simulink model "MODELL_aktiver_Stabi"  (R2016a)
settings: Solver=ode4  StartTime=0.0  StopTime=10  FixedStep=0.001  RelTol=1e-3
undefined symbols (not defined in the file): A_Kolben, b_d, b_f, b_r, b_s, c, c_R, d, d_R, G, g, h_Aktor, h_S_DZ, h_Stabi, I_p_Stabi, J_x_A, J_x_F, m_A, m_F, m_R, sigbuilder_block
settings Model: Creator=Michaél  LastModifiedBy=Michaél

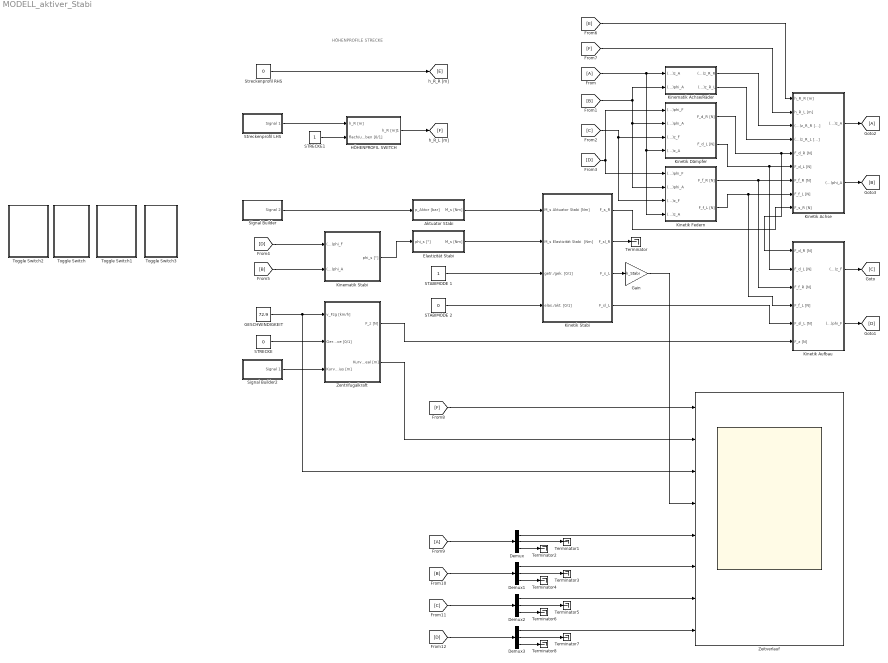
== system MODELL_aktiver_Stabi ==
  note: HÖHENPROFILE
      | STRECKE
  Aktuator Stabi : Subsystem
  Demux{,1..3} (4 alike) : Demux  Outputs=3
  Elastizität Stabi : Subsystem
  GESCHWINDIGKEIT : Constant  Value=72.9
  Gain : Gain  Gain=h_Stabi
  HÖHENPROFIL SWITCH : Subsystem
  Kinematik Achse/Räder : Subsystem
  Kinematik Stabi : Subsystem
  Kinetik Achse : Subsystem
  Kinetik Aufbau : Subsystem
  Kinetik Dämpfer : Subsystem
  Kinetik Federn : Subsystem
  Kinetik Stabi : Subsystem
  STABIMODE 1 : Constant
  STABIMODE 2 : Constant  Value=0
  STRECKE : Constant  Value=0
  STRECKE1 : Constant
  Signal Builder : Subsystem  Tag=STV Subsys  LoadFcn=sigbuilder_block('load');  StartFcn=sigbuilder_block('start');  StopFcn=sigbuilder_block('stop');  ClipboardFcn=sigbuilder_block('clipboard');  mask(Sigbuilder block){}
      mask help: Simulink:masks:SigbuilderBlock_MD
      mask init:
      | if ~strcmp(get_param(bdroot(gcbh),'SimulationStatus'),'stopped') tuvar = sigbuilder_block('maskInit'); end
      settings: CopyFcn=sigbuilder_block('copy');  DeleteFcn=sigbuilder_block('delete');  ModelCloseFcn=sigbuilder_block('modelClose');  PreSaveFcn=sigbuilder_block('preSave');  PauseFcn=sigbuilder_block('pause');  ContinueFcn=sigbuilder_block('continue');  NameChangeFcn=sigbuilder_block('namechange');  OpenFcn=sigbuilder_block('open',[437.25 153 550.5 359.25 ]);  CloseFcn=sigbuilder_block('close');
      mask Display: plot(0, 0, 100, 100,[2, 2, 32, 32, 2], [68, 8, 8, 68, 68],[32, 2], [38, 38], [32, 19, 2],[53, 60, 44], [32, 17, 17, 2],[16, 16, 31, 31]);txt = getActiveGroup(gcbh);text(2, 100, txt,'verticalAlignment', 'top');
  Signal Builder2 : Subsystem  Tag=STV Subsys  LoadFcn=sigbuilder_block('load');  StartFcn=sigbuilder_block('start');  StopFcn=sigbuilder_block('stop');  ClipboardFcn=sigbuilder_block('clipboard');  mask(Sigbuilder block){}
      mask help: Simulink:masks:SigbuilderBlock_MD
      mask init:
      | if ~strcmp(get_param(bdroot(gcbh),'SimulationStatus'),'stopped') tuvar = sigbuilder_block('maskInit'); end
      settings: CopyFcn=sigbuilder_block('copy');  DeleteFcn=sigbuilder_block('delete');  ModelCloseFcn=sigbuilder_block('modelClose');  PreSaveFcn=sigbuilder_block('preSave');  PauseFcn=sigbuilder_block('pause');  ContinueFcn=sigbuilder_block('continue');  NameChangeFcn=sigbuilder_block('namechange');  OpenFcn=sigbuilder_block('open',[437.25 153 550.5 359.25 ]);  CloseFcn=sigbuilder_block('close');
      mask Display: plot(0, 0, 100, 100,[2, 2, 32, 32, 2], [68, 8, 8, 68, 68],[32, 2], [38, 38], [32, 19, 2],[53, 60, 44], [32, 17, 17, 2],[16, 16, 31, 31]);txt = getActiveGroup(gcbh);text(2, 100, txt,'verticalAlignment', 'top');
  Streckenprofil LHS : Subsystem  Tag=STV Subsys  LoadFcn=sigbuilder_block('load');  StartFcn=sigbuilder_block('start');  StopFcn=sigbuilder_block('stop');  ClipboardFcn=sigbuilder_block('clipboard');  mask(Sigbuilder block){}
      mask help: Simulink:masks:SigbuilderBlock_MD
      mask init:
      | if ~strcmp(get_param(bdroot(gcbh),'SimulationStatus'),'stopped') tuvar = sigbuilder_block('maskInit'); end
      settings: CopyFcn=sigbuilder_block('copy');  DeleteFcn=sigbuilder_block('delete');  ModelCloseFcn=sigbuilder_block('modelClose');  PreSaveFcn=sigbuilder_block('preSave');  PauseFcn=sigbuilder_block('pause');  ContinueFcn=sigbuilder_block('continue');  NameChangeFcn=sigbuilder_block('namechange');  OpenFcn=sigbuilder_block('open',[437.25 153 550.5 359.25 ]);  CloseFcn=sigbuilder_block('close');
      mask Display: plot(0, 0, 100, 100,[2, 2, 32, 32, 2], [68, 8, 8, 68, 68],[32, 2], [38, 38], [32, 19, 2],[53, 60, 44], [32, 17, 17, 2],[16, 16, 31, 31]);txt = getActiveGroup(gcbh);text(2, 100, txt,'verticalAlignment', 'top');
  Streckenprofil RHS : Constant  Value=0
  Terminator{,1..8} (9 alike) : Terminator
  Toggle Switch : Subsystem  DialogController=hmiCreateDDGDialog  IsWebBlock=on  mask(MWDashboardBlock){webBlockId=3030378f-6338-4f5a-b9a6-65f9c6752063, webBlockType=toggleswitch, ShowInLibBrowser=on, ShowInitialText=on, HMISrcModelName=MODELL_aktiver_Stabi_OPENME}
      mask prompts: webBlockId "WebBlock Id"; webBlockType "WebBlock Type"; HMISrcModelName "Source Model"
      mask help: Set on/off value to tune parameters or variables.
      mask Help: helpview([docroot '/mapfiles/simulink.map'], 'hmi_switch')
      mask Display:
      | if strcmp(get_param(bdroot(gcb),'BlockDiagramType'),'library')
      |  image([(matlabroot) '/toolbox/simulink/hmi/icons/ToggleSwitch.png'])
      | end
  Toggle Switch1 : Subsystem  DialogController=hmiCreateDDGDialog  IsWebBlock=on  mask(MWDashboardBlock){webBlockId=66d0c5f1-b412-4773-8f90-b24a010b2d54, webBlockType=toggleswitch, ShowInLibBrowser=on, ShowInitialText=on, HMISrcModelName=MODELL_aktiver_Stabi_OPENME}
      mask prompts: webBlockId "WebBlock Id"; webBlockType "WebBlock Type"; HMISrcModelName "Source Model"
      mask help: Set on/off value to tune parameters or variables.
      mask Help: helpview([docroot '/mapfiles/simulink.map'], 'hmi_switch')
      mask Display:
      | if strcmp(get_param(bdroot(gcb),'BlockDiagramType'),'library')
      |  image([(matlabroot) '/toolbox/simulink/hmi/icons/ToggleSwitch.png'])
      | end
  Toggle Switch2 : Subsystem  DialogController=hmiCreateDDGDialog  IsWebBlock=on  mask(MWDashboardBlock){webBlockId=f8bafa90-b455-434b-b4c4-d0f007b97158, webBlockType=toggleswitch, ShowInLibBrowser=on, ShowInitialText=on, HMISrcModelName=MODELL_aktiver_Stabi_OPENME}
      mask prompts: webBlockId "WebBlock Id"; webBlockType "WebBlock Type"; HMISrcModelName "Source Model"
      mask help: Set on/off value to tune parameters or variables.
      mask Help: helpview([docroot '/mapfiles/simulink.map'], 'hmi_switch')
      mask Display:
      | if strcmp(get_param(bdroot(gcb),'BlockDiagramType'),'library')
      |  image([(matlabroot) '/toolbox/simulink/hmi/icons/ToggleSwitch.png'])
      | end
  Toggle Switch3 : Subsystem  DialogController=hmiCreateDDGDialog  IsWebBlock=on  mask(MWDashboardBlock){webBlockId=5b0afa38-ed08-4fc5-84e4-437145695883, webBlockType=toggleswitch, ShowInLibBrowser=on, ShowInitialText=on, HMISrcModelName=MODELL_aktiver_Stabi_OPENME}
      mask prompts: webBlockId "WebBlock Id"; webBlockType "WebBlock Type"; HMISrcModelName "Source Model"
      mask help: Set on/off value to tune parameters or variables.
      mask Help: helpview([docroot '/mapfiles/simulink.map'], 'hmi_switch')
      mask Display:
      | if strcmp(get_param(bdroot(gcb),'BlockDiagramType'),'library')
      |  image([(matlabroot) '/toolbox/simulink/hmi/icons/ToggleSwitch.png'])
      | end
  Zeitverlauf : Scope  NumInputPorts=8
  Zentrifugalkraft : Subsystem
  wires:
  Aktuator Stabi/1(M_s [Nm]) -> Kinetik Stabi/1(M_s Aktuator Stabi [Nm])
  Kinetik Stabi/2(F_sl_R) -> Terminator/1
  Kinetik Federn/1(F_f_R [N]) -> Kinetik Aufbau/3(F_f_R [N]), Kinetik Achse/7(F_f_R [N])
  Kinetik Federn/2(F_f_L [N]) -> Kinetik Aufbau/4(F_f_L [N]), Kinetik Achse/8(F_f_L [N])
  Kinetik Dämpfer/1(F_d_R [N]) -> Kinetik Aufbau/1(F_d_R [N]), Kinetik Achse/5(F_d_R [N])
  Kinetik Dämpfer/2(F_d_L [N]) -> Kinetik Aufbau/2(F_d_L [N]), Kinetik Achse/6(F_d_L [N])
  Kinetik Stabi/3(F_s_L) -> Gain/1
  Zentrifugalkraft/1(F_z [N]) -> Kinetik Aufbau/6("F_z [N] ")
  Kinematik Stabi/1(phi_s [°]) -> Elastizität Stabi/1(phi_s [°])
  Kinematik Achse/Räder/1((...)z_R_R) -> Kinetik Achse/3((...)z_R_R [...])
  Kinematik Achse/Räder/2((...)z_R_L) -> Kinetik Achse/4((...)z_R_L [...])
  Kinetik Aufbau/1((...)z_F) -> [C]
  Kinetik Aufbau/2((...)phi_F) -> [D]
  Kinetik Achse/1((...)z_A) -> [A]
  Kinetik Achse/2((...)phi_A) -> [B]
  [A] -> Kinetik Federn/4((...)z_A), Kinetik Dämpfer/4((...)z_A), Kinematik Achse/Räder/1((...)z_A)
  [B] -> Kinetik Federn/2((...)phi_A), Kinetik Dämpfer/2((...)phi_A), Kinematik Achse/Räder/2((...)phi_A)
  [C] -> Kinetik Dämpfer/3((...)z_F), Kinetik Federn/3((...)z_F)
  [D] -> Kinetik Federn/1((...)phi_F), Kinetik Dämpfer/1((...)phi_F)
  [D] -> Kinematik Stabi/1((...)phi_F)
  [B] -> Kinematik Stabi/2((...)phi_A)
  STABIMODE 1/1 -> Kinetik Stabi/3("getr./gek. [0/1] ")
  STRECKE/1 -> Zentrifugalkraft/2(Gerade/Kurve [0/1])
  STABIMODE 2/1 -> Kinetik Stabi/4("elas./akt. [0/1] ")
  [E] -> Kinetik Achse/1(h_R_R [m])
  [F] -> Kinetik Achse/2(h_R_L [m])
  Signal Builder/1(Signal 2) -> Aktuator Stabi/1(p_Aktor [bar])
  Signal Builder2/1(Signal 1) -> Zentrifugalkraft/3(Kurvenradius [m])
  [F] -> Zeitverlauf/1
  GESCHWINDIGKEIT/1 -> Zeitverlauf/3, Zentrifugalkraft/1(v_Fzg [km/h])
  [A] -> Demux/1
  Demux/1 -> Zeitverlauf/5
  [B] -> Demux1/1
  Demux1/1 -> Zeitverlauf/6
  [C] -> Demux2/1
  Demux2/1 -> Zeitverlauf/7
  [D] -> Demux3/1
  Elastizität Stabi/1(M_s [Nm]) -> Kinetik Stabi/2(M_s Elastizität Stabi  [Nm])
  Gain/1 -> Zeitverlauf/4
  Kinetik Stabi/1(F_s_R) -> Kinetik Achse/9(F_s_R [N])
  Kinetik Stabi/4(F_sl_L) -> Kinetik Aufbau/5("F_sl_L [N] ")
  Streckenprofil RHS/1 -> [E]
  Streckenprofil LHS/1(Signal 1) -> HÖHENPROFIL SWITCH/1(h_R [m])
  HÖHENPROFIL SWITCH/1(h_R [m]1) -> [F]
  STRECKE1/1 -> HÖHENPROFIL SWITCH/2(flach/uneben [0/1])
  Demux3/1 -> Zeitverlauf/8
  Demux/2 -> Terminator1/1
  Demux/3 -> Terminator2/1
  Demux1/2 -> Terminator3/1
  Demux1/3 -> Terminator4/1
  Demux2/2 -> Terminator5/1
  Demux2/3 -> Terminator6/1
  Demux3/2 -> Terminator7/1
  Demux3/3 -> Terminator8/1
  Zentrifugalkraft/2(Kurvenradius real [m]) -> Zeitverlauf/2

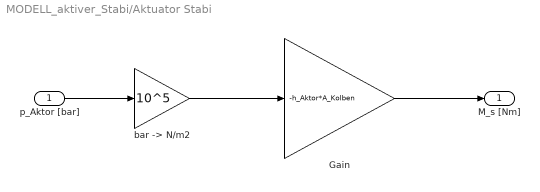
== system MODELL_aktiver_Stabi/Aktuator Stabi ==
  p_Aktor [bar] : Inport
  Gain : Gain  Gain=-h_Aktor*A_Kolben
  "bar -> N/m2" : Gain  Gain=10^5
  M_s [Nm] : Outport
  wires:
  Gain/1 -> M_s [Nm]/1
  p_Aktor [bar]/1 -> "bar -> N/m2"/1
  "bar -> N/m2"/1 -> Gain/1

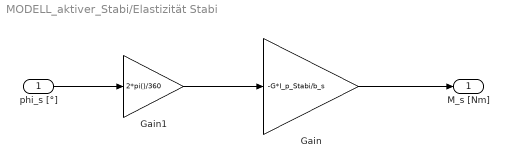
== system MODELL_aktiver_Stabi/Elastizität Stabi ==
  phi_s [°] : Inport
  Gain : Gain  Gain=-G*I_p_Stabi/b_s
  Gain1 : Gain  Gain=2*pi()/360
  M_s [Nm] : Outport
  wires:
  phi_s [°]/1 -> Gain1/1
  Gain1/1 -> Gain/1
  Gain/1 -> M_s [Nm]/1

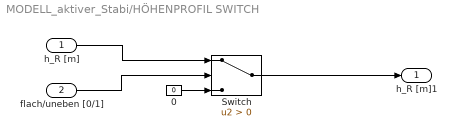
== system MODELL_aktiver_Stabi/HÖHENPROFIL SWITCH ==
  h_R [m] : Inport
  flach/uneben [0/1] : Inport  Port=2
  0 : Constant  Value=0
  Switch : Switch  Criteria=u2 > Threshold
  h_R [m]1 : Outport
  wires:
  h_R [m]/1 -> Switch/1
  Switch/1 -> h_R [m]1/1
  flach/uneben [0/1]/1 -> Switch/2
  0/1 -> Switch/3

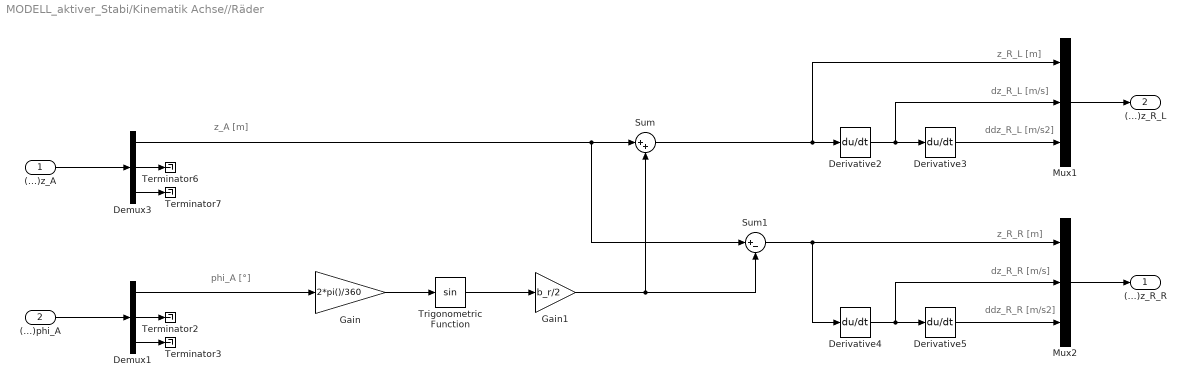
== system MODELL_aktiver_Stabi/Kinematik Achse//Räder ==
  note: z_R_L [m]
  note: dz_R_L [m/s]
  note: ddz_R_L [m/s2]
  note: z_R_R [m]
  note: dz_R_R [m/s]
  note: ddz_R_R [m/s2]
  note: z_A [m]
  note: phi_A [°]
  (...)z_A : Inport
  (...)phi_A : Inport  Port=2
  Demux1 : Demux  Outputs=3
  Demux3 : Demux  Outputs=3
  Derivative{2..5} (4 alike) : Derivative
  Gain : Gain  Gain=2*pi()/360
  Gain1 : Gain  Gain=b_r/2
  Mux1 : Mux  Inputs=3
  Mux2 : Mux  Inputs=3
  Sum : Sum  Inputs=|++
  Sum1 : Sum  Inputs=|+-
  Terminator{2..3,6..7} (4 alike) : Terminator
  Trigonometric Function : Trigonometry
  (...)z_R_R : Outport
  (...)z_R_L : Outport  Port=2
  wires:
  Gain/1 -> Trigonometric Function/1
  Trigonometric Function/1 -> Gain1/1
  Demux1/1 -> Gain/1
  Demux3/1 -> Sum1/1, Sum/1
  Gain1/1 -> Sum1/2, Sum/2
  Derivative3/1 -> Mux1/3
  Derivative2/1 -> Mux1/2, Derivative3/1
  Sum/1 -> Mux1/1, Derivative2/1
  Mux1/1 -> (...)z_R_L/1
  Derivative5/1 -> Mux2/3
  Derivative4/1 -> Mux2/2, Derivative5/1
  Sum1/1 -> Derivative4/1, Mux2/1
  Mux2/1 -> (...)z_R_R/1
  (...)z_A/1 -> Demux3/1
  Demux3/3 -> Terminator7/1
  Demux3/2 -> Terminator6/1
  (...)phi_A/1 -> Demux1/1
  Demux1/3 -> Terminator3/1
  Demux1/2 -> Terminator2/1

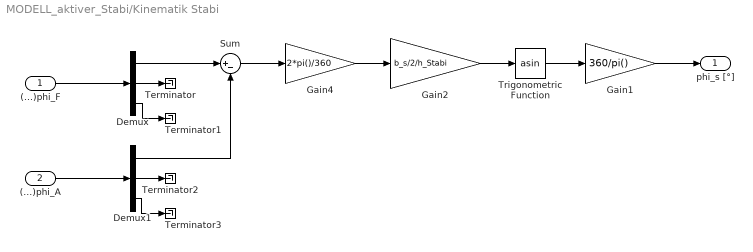
== system MODELL_aktiver_Stabi/Kinematik Stabi ==
  (...)phi_F : Inport
  (...)phi_A : Inport  Port=2
  Demux : Demux  Outputs=3
  Demux1 : Demux  Outputs=3
  Gain1 : Gain  Gain=360/pi()
  Gain2 : Gain  Gain=b_s/2/h_Stabi
  Gain4 : Gain  Gain=2*pi()/360
  Sum : Sum  Inputs=|+-
  Terminator{,1..3} (4 alike) : Terminator
  Trigonometric Function : Trigonometry  Operator=asin
  phi_s [°] : Outport
  wires:
  Sum/1 -> Gain4/1
  (...)phi_F/1 -> Demux/1
  (...)phi_A/1 -> Demux1/1
  Demux/1 -> Sum/1
  Demux1/1 -> Sum/2
  Demux/2 -> Terminator/1
  Demux/3 -> Terminator1/1
  Demux1/3 -> Terminator3/1
  Demux1/2 -> Terminator2/1
  Gain2/1 -> Trigonometric Function/1
  Gain1/1 -> phi_s [°]/1
  Gain4/1 -> Gain2/1
  Trigonometric Function/1 -> Gain1/1

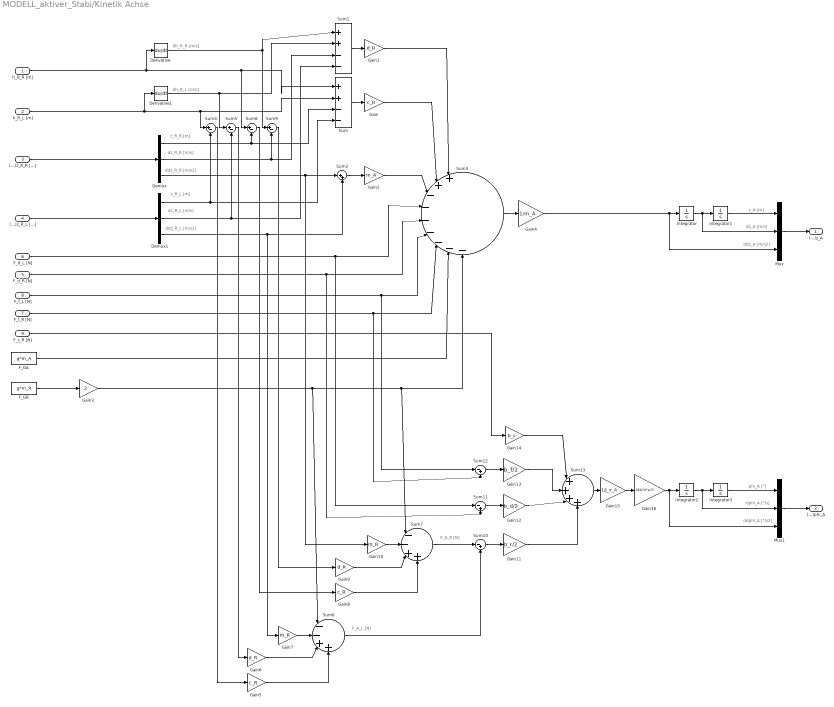
== system MODELL_aktiver_Stabi/Kinetik Achse ==
  note: F_A_L [N]
  note: dh_R_L [m/s]
  note: dh_R_R [m/s]
  note: z_R_L [m]
  note: dz_R_L [m/s]
  note: ddz_R_L [m/s2]
  note: z_R_R [m]
  note: dz_R_R [m/s]
  note: ddz_R_R [m/s2]
  note: z_A [m]
  note: dz_A [m/s]
  note: ddz_A [m/s2]
  note: F_A_R [N]
  note: phi_A [°]
  note: dphi_A [°/s]
  note: ddphi_A [°/s2]
  h_R_R [m] : Inport
  h_R_L [m] : Inport  Port=2
  (...)z_R_R [...] : Inport  Port=3
  (...)z_R_L [...] : Inport  Port=4
  F_d_R [N] : Inport  Port=5
  F_d_L [N] : Inport  Port=6
  F_f_R [N] : Inport  Port=7
  F_f_L [N] : Inport  Port=8
  F_s_R [N] : Inport  Port=9
  Demux : Demux  Outputs=3
  Demux1 : Demux  Outputs=3
  Derivative : Derivative
  Derivative1 : Derivative
  F_GA : Constant  Value=g*m_A
  F_GR : Constant  Value=g*m_R
  Gain : Gain  Gain=c_R
  Gain1 : Gain  Gain=d_R
  Gain10 : Gain  Gain=m_R
  Gain11 : Gain  Gain=b_r/2
  Gain12 : Gain  Gain=b_d/2
  Gain13 : Gain  Gain=b_f/2
  Gain14 : Gain  Gain=b_s
  Gain15 : Gain  Gain=1/J_x_A
  Gain16 : Gain  Gain=360/(2*pi())
  Gain2 : Gain  Gain=m_A
  Gain3 : Gain  Gain=2
  Gain4 : Gain  Gain=1/m_A
  Gain5 : Gain  Gain=c_R
  Gain6 : Gain  Gain=d_R
  Gain7 : Gain  Gain=m_R
  Gain8 : Gain  Gain=c_R
  Gain9 : Gain  Gain=d_R
  Integrator : Integrator
  Integrator1 : Integrator  InitialCondition=-0.03
  Integrator2 : Integrator
  Integrator3 : Integrator
  Mux : Mux  Inputs=3
  Mux1 : Mux  Inputs=3
  Sum : Sum  Inputs=|++--
  Sum1 : Sum  Inputs=|++--
  Sum10 : Sum  Inputs=|-+
  Sum11 : Sum  Inputs=|-+
  Sum12 : Sum  Inputs=|-+
  Sum13 : Sum  Inputs=|++++
  Sum2 : Sum  Inputs=|++
  Sum3 : Sum  Inputs=|++-------
  Sum{4..5,8..9} (4 alike) : Sum  Inputs=|+-
  Sum6 : Sum  Inputs=|--++
  Sum7 : Sum  Inputs=|--++
  (...)z_A : Outport
  (...)phi_A : Outport  Port=2
  wires:
  (...)z_R_R [...]/1 -> Demux/1
  (...)z_R_L [...]/1 -> Demux1/1
  h_R_R [m]/1 -> Sum8/1, Sum/1, Derivative/1
  h_R_L [m]/1 -> Sum4/1, Sum/2, Derivative1/1
  Demux/1 -> Sum8/2, Sum/3
  Demux1/1 -> Sum/4, Sum4/2
  Sum/1 -> Gain/1
  Derivative/1 -> Sum9/1, Sum1/1
  Derivative1/1 -> Sum1/2, Sum5/1
  Demux1/2 -> Sum1/4, Sum5/2
  Demux1/3 -> Sum2/2, Gain7/1
  Sum1/1 -> Gain1/1
  Sum2/1 -> Gain2/1
  F_GR/1 -> Gain3/1
  Gain1/1 -> Sum3/1
  Gain/1 -> Sum3/2
  Gain2/1 -> Sum3/3
  F_d_R [N]/1 -> Sum3/5, Sum11/2
  F_f_L [N]/1 -> Sum12/1, Sum3/6
  F_GA/1 -> Sum3/8
  Gain3/1 -> Sum3/9, Sum7/1, Sum6/1
  Sum3/1 -> Gain4/1
  Gain4/1 -> Mux/3, Integrator/1
  Integrator/1 -> Mux/2, Integrator1/1
  Integrator1/1 -> Mux/1
  Mux/1 -> (...)z_A/1
  Sum4/1 -> Gain5/1
  Sum5/1 -> Gain6/1
  Gain5/1 -> Sum6/4
  Gain6/1 -> Sum6/3
  Gain7/1 -> Sum6/2
  Demux/3 -> Gain10/1, Sum2/1
  Sum8/1 -> Gain8/1
  Sum9/1 -> Gain9/1
  Gain8/1 -> Sum7/4
  Gain9/1 -> Sum7/3
  Gain10/1 -> Sum7/2
  Demux/2 -> Sum9/2, Sum1/3
  Sum7/1 -> Sum10/1
  Sum6/1 -> Sum10/2
  Sum10/1 -> Gain11/1
  F_d_L [N]/1 -> Sum11/1, Sum3/4
  Sum11/1 -> Gain12/1
  F_f_R [N]/1 -> Sum12/2, Sum3/7
  Sum12/1 -> Gain13/1
  F_s_R [N]/1 -> Gain14/1
  Gain14/1 -> Sum13/1
  Gain13/1 -> Sum13/2
  Gain12/1 -> Sum13/3
  Gain11/1 -> Sum13/4
  Sum13/1 -> Gain15/1
  Gain15/1 -> Gain16/1
  Integrator2/1 -> Mux1/2, Integrator3/1
  Integrator3/1 -> Mux1/1
  Mux1/1 -> (...)phi_A/1
  Gain16/1 -> Mux1/3, Integrator2/1

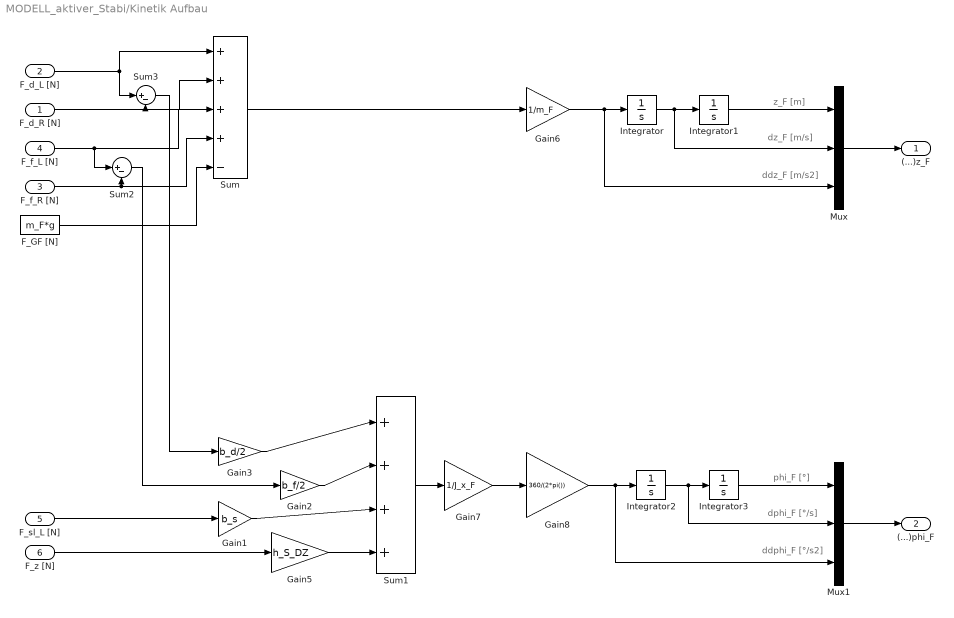
== system MODELL_aktiver_Stabi/Kinetik Aufbau ==
  note: z_F [m]
  note: dz_F [m/s]
  note: ddz_F [m/s2]
  note: phi_F [°]
  note: dphi_F [°/s]
  note: ddphi_F [°/s2]
  F_d_R [N] : Inport
  F_d_L [N] : Inport  Port=2
  F_f_R [N] : Inport  Port=3
  F_f_L [N] : Inport  Port=4
  "F_sl_L [N] " : Inport  Port=5
  "F_z [N] " : Inport  Port=6
  F_GF [N] : Constant  Value=m_F*g
  Gain1 : Gain  Gain=b_s
  Gain2 : Gain  Gain=b_f/2
  Gain3 : Gain  Gain=b_d/2
  Gain5 : Gain  Gain=h_S_DZ
  Gain6 : Gain  Gain=1/m_F
  Gain7 : Gain  Gain=1/J_x_F
  Gain8 : Gain  Gain=360/(2*pi())
  Integrator : Integrator
  Integrator1 : Integrator  InitialCondition=-0.15
  Integrator2 : Integrator
  Integrator3 : Integrator
  Mux : Mux  Inputs=3
  Mux1 : Mux  Inputs=3
  Sum : Sum  Inputs=|++++-
  Sum1 : Sum  Inputs=|++++
  Sum2 : Sum  Inputs=|+-
  Sum3 : Sum  Inputs=|+-
  (...)z_F : Outport
  (...)phi_F : Outport  Port=2
  wires:
  F_d_L [N]/1 -> Sum3/1, Sum/1
  F_d_R [N]/1 -> Sum/2, Sum3/2
  F_f_L [N]/1 -> Sum2/1, Sum/3
  F_f_R [N]/1 -> Sum/4, Sum2/2
  F_GF [N]/1 -> Sum/5
  Sum/1 -> Gain6/1
  Gain6/1 -> Mux/3, Integrator/1
  Integrator/1 -> Mux/2, Integrator1/1
  "F_sl_L [N] "/1 -> Gain1/1
  Gain1/1 -> Sum1/3
  Sum2/1 -> Gain2/1
  Gain2/1 -> Sum1/2
  Gain3/1 -> Sum1/1
  Sum3/1 -> Gain3/1
  Gain5/1 -> Sum1/4
  "F_z [N] "/1 -> Gain5/1
  Sum1/1 -> Gain7/1
  Gain7/1 -> Gain8/1
  Integrator1/1 -> Mux/1
  Mux/1 -> (...)z_F/1
  Gain8/1 -> Mux1/3, Integrator2/1
  Integrator2/1 -> Mux1/2, Integrator3/1
  Integrator3/1 -> Mux1/1
  Mux1/1 -> (...)phi_F/1

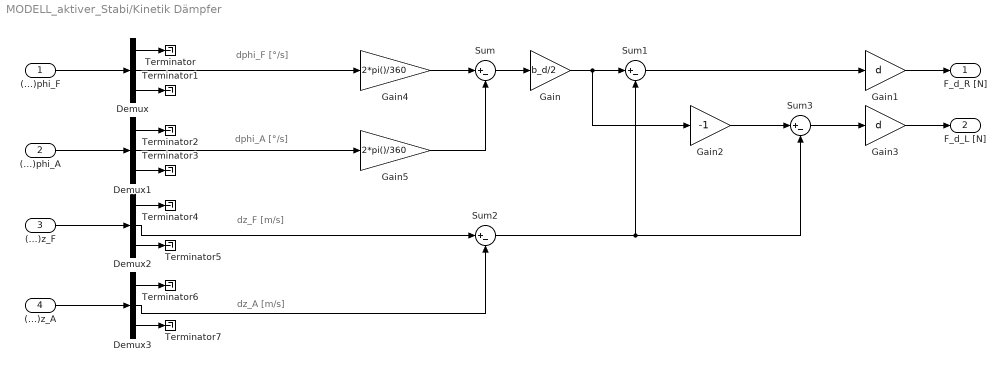
== system MODELL_aktiver_Stabi/Kinetik Dämpfer ==
  note: dz_A [m/s]
  note: dphi_A [°/s]
  note: dphi_F [°/s]
  note: dz_F [m/s]
  (...)phi_F : Inport
  (...)phi_A : Inport  Port=2
  (...)z_F : Inport  Port=3
  (...)z_A : Inport  Port=4
  Demux{,1..3} (4 alike) : Demux  Outputs=3
  Gain : Gain  Gain=b_d/2
  Gain1 : Gain  Gain=d
  Gain2 : Gain  Gain=-1
  Gain3 : Gain  Gain=d
  Gain4 : Gain  Gain=2*pi()/360
  Gain5 : Gain  Gain=2*pi()/360
  Sum{,1..3} (4 alike) : Sum  Inputs=|+-
  Terminator{,1..7} (8 alike) : Terminator
  F_d_R [N] : Outport
  F_d_L [N] : Outport  Port=2
  wires:
  Demux/2 -> Gain4/1
  Demux1/2 -> Gain5/1
  Sum/1 -> Gain/1
  Gain/1 -> Gain2/1, Sum1/1
  Demux2/2 -> Sum2/1
  Demux3/2 -> Sum2/2
  Sum2/1 -> Sum1/2, Sum3/2
  Sum1/1 -> Gain1/1
  Gain1/1 -> F_d_R [N]/1
  Gain2/1 -> Sum3/1
  Gain3/1 -> F_d_L [N]/1
  Sum3/1 -> Gain3/1
  Gain4/1 -> Sum/1
  Gain5/1 -> Sum/2
  (...)phi_F/1 -> Demux/1
  (...)phi_A/1 -> Demux1/1
  Demux/3 -> Terminator1/1
  Demux1/3 -> Terminator3/1
  Demux/1 -> Terminator/1
  Demux1/1 -> Terminator2/1
  (...)z_F/1 -> Demux2/1
  (...)z_A/1 -> Demux3/1
  Demux2/3 -> Terminator5/1
  Demux3/3 -> Terminator7/1
  Demux2/1 -> Terminator4/1
  Demux3/1 -> Terminator6/1

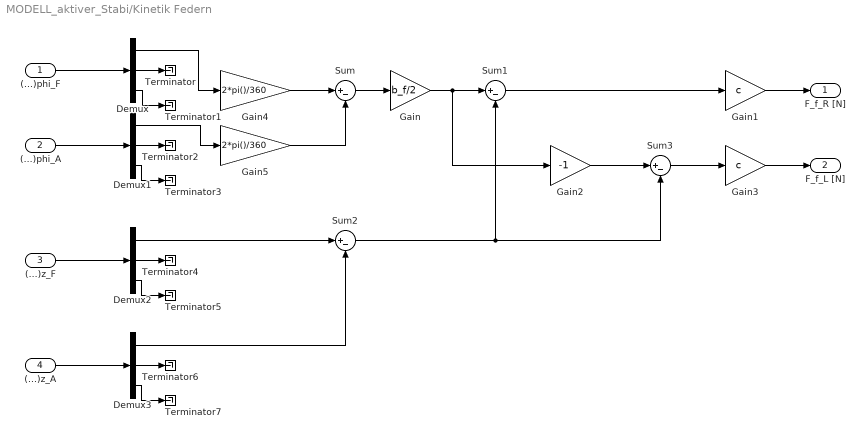
== system MODELL_aktiver_Stabi/Kinetik Federn ==
  (...)phi_F : Inport
  (...)phi_A : Inport  Port=2
  (...)z_F : Inport  Port=3
  (...)z_A : Inport  Port=4
  Demux{,1..3} (4 alike) : Demux  Outputs=3
  Gain : Gain  Gain=b_f/2
  Gain1 : Gain  Gain=c
  Gain2 : Gain  Gain=-1
  Gain3 : Gain  Gain=c
  Gain4 : Gain  Gain=2*pi()/360
  Gain5 : Gain  Gain=2*pi()/360
  Sum{,1..3} (4 alike) : Sum  Inputs=|+-
  Terminator{,1..7} (8 alike) : Terminator
  F_f_R [N] : Outport
  F_f_L [N] : Outport  Port=2
  wires:
  (...)phi_F/1 -> Demux/1
  (...)phi_A/1 -> Demux1/1
  Sum/1 -> Gain/1
  Gain/1 -> Gain2/1, Sum1/1
  Sum2/1 -> Sum3/2, Sum1/2
  Sum1/1 -> Gain1/1
  Gain1/1 -> F_f_R [N]/1
  Gain2/1 -> Sum3/1
  Gain3/1 -> F_f_L [N]/1
  Sum3/1 -> Gain3/1
  Gain4/1 -> Sum/1
  Gain5/1 -> Sum/2
  Demux/1 -> Gain4/1
  Demux1/1 -> Gain5/1
  Demux/2 -> Terminator/1
  Demux/3 -> Terminator1/1
  Demux1/3 -> Terminator3/1
  Demux1/2 -> Terminator2/1
  (...)z_F/1 -> Demux2/1
  Demux2/3 -> Terminator5/1
  Demux2/2 -> Terminator4/1
  Demux2/1 -> Sum2/1
  (...)z_A/1 -> Demux3/1
  Demux3/3 -> Terminator7/1
  Demux3/2 -> Terminator6/1
  Demux3/1 -> Sum2/2

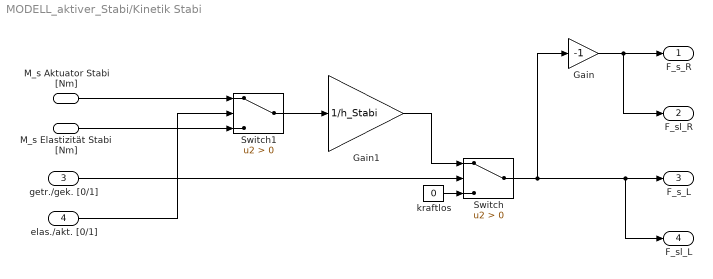
== system MODELL_aktiver_Stabi/Kinetik Stabi ==
  M_s Aktuator Stabi [Nm] : Inport
  M_s Elastizität Stabi  [Nm] : Inport  Port=2
  "getr./gek. [0/1] " : Inport  Port=3
  "elas./akt. [0/1] " : Inport  Port=4
  Gain : Gain  Gain=-1
  Gain1 : Gain  Gain=1/h_Stabi
  Switch : Switch  Criteria=u2 > Threshold
  Switch1 : Switch  Criteria=u2 > Threshold
  kraftlos : Constant  Value=0
  F_s_R : Outport
  F_sl_R : Outport  Port=2
  F_s_L : Outport  Port=3
  F_sl_L : Outport  Port=4
  wires:
  Gain/1 -> F_sl_R/1, F_s_R/1
  Switch/1 -> Gain/1, F_sl_L/1, F_s_L/1
  "getr./gek. [0/1] "/1 -> Switch/2
  Gain1/1 -> Switch/1
  kraftlos/1 -> Switch/3
  Switch1/1 -> Gain1/1
  M_s Aktuator Stabi [Nm]/1 -> Switch1/1
  M_s Elastizität Stabi  [Nm]/1 -> Switch1/3
  "elas./akt. [0/1] "/1 -> Switch1/2

== system MODELL_aktiver_Stabi/Signal Builder ==
  Demux : Demux  Tag=STV Demux  Outputs=1
  FromWs : FromWorkspace  Tag=STV FromWs  VariableName=tuvar  SampleTime=0
      SigBuilderData=|
      | common.afterFinalStr = 'Extrapolate'
      | common.sampleTime = 0
      | dataSet.timeRange = [0 10]
      | dataSet.name = 'Group 1'
      | sbobj.Groups.Name = 'Group 1'
      | sbobj.Groups.Signals.Name = 'Signal 2'
      | sbobj.Groups.Signals.XData = [0 2 2 4 4 10]
      | sbobj.Groups.Signals.YData = [0 0 10 10 0 0]
  Signal 2 : Outport  Tag=STV Outport
  wires:
  FromWs/1 -> Demux/1
  Demux/1 -> Signal 2/1

== system MODELL_aktiver_Stabi/Signal Builder2 ==
  Demux : Demux  Tag=STV Demux  Outputs=1
  FromWs : FromWorkspace  Tag=STV FromWs  VariableName=tuvar  SampleTime=0
      SigBuilderData=|
      | common.afterFinalStr = 'Extrapolate'
      | common.sampleTime = 0
      | dataSet.timeRange = [0 10]
      | dataSet.name = 'Group 1'
      | sbobj.Groups.Name = 'Group 1'
      | sbobj.Groups.Signals.Name = 'Signal 1'
      | sbobj.Groups.Signals.XData = [0 1 2 2 4.5 5.5 10]
      | sbobj.Groups.Signals.YData = [1000 1000 12 12.5 12.5 1000 1000]
  Signal 1 : Outport  Tag=STV Outport
  wires:
  Demux/1 -> Signal 1/1
  FromWs/1 -> Demux/1

== system MODELL_aktiver_Stabi/Streckenprofil LHS ==
  Demux : Demux  Tag=STV Demux  Outputs=1
  FromWs : FromWorkspace  Tag=STV FromWs  VariableName=tuvar  SampleTime=0
      SigBuilderData=|
      | common.afterFinalStr = 'Extrapolate'
      | common.sampleTime = 0
      | dataSet.timeRange = [0 10]
      | dataSet.name = 'Group 1'
      | sbobj.Groups.Name = 'Group 1'
      | sbobj.Groups.Signals.Name = 'Signal 1'
      | sbobj.Groups.Signals.XData = [0 7 7.025 7.05 10]
      | sbobj.Groups.Signals.YData = [0 0 -0.04 0 0]
  Signal 1 : Outport  Tag=STV Outport
  wires:
  Demux/1 -> Signal 1/1
  FromWs/1 -> Demux/1

== system MODELL_aktiver_Stabi/Toggle Switch ==

== system MODELL_aktiver_Stabi/Toggle Switch1 ==

== system MODELL_aktiver_Stabi/Toggle Switch2 ==

== system MODELL_aktiver_Stabi/Toggle Switch3 ==

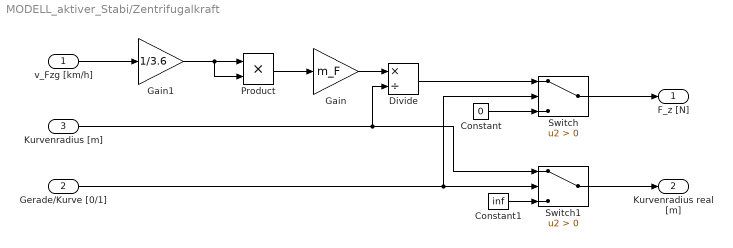
== system MODELL_aktiver_Stabi/Zentrifugalkraft ==
  v_Fzg [km/h] : Inport
  Gerade/Kurve [0/1] : Inport  Port=2
  Kurvenradius [m] : Inport  Port=3
  Constant : Constant  Value=0
  Constant1 : Constant  Value=inf
  Divide : Product  Inputs=*/
  Gain : Gain  Gain=m_F
  Gain1 : Gain  Gain=1/3.6
  Product : Product
  Switch : Switch  Criteria=u2 > Threshold
  Switch1 : Switch  Criteria=u2 > Threshold
  F_z [N] : Outport
  Kurvenradius real [m] : Outport  Port=2
  wires:
  v_Fzg [km/h]/1 -> Gain1/1
  Product/1 -> Gain/1
  Gain/1 -> Divide/1
  Switch/1 -> F_z [N]/1
  Constant/1 -> Switch/3
  Gerade/Kurve [0/1]/1 -> Switch/2, Switch1/2
  Gain1/1 -> Product/2, Product/1
  Divide/1 -> Switch/1
  Kurvenradius [m]/1 -> Switch1/1, Divide/2
  Constant1/1 -> Switch1/3
  Switch1/1 -> Kurvenradius real [m]/1
